simulink library "dtcBswLib"  (R2023b)
settings: Solver=VariableStepAuto  StartTime=0.0  StopTime=10.0  RelTol=1e-3
libraries: dtc_bswapi x5, simulink x2
settings Model: Creator=Professional  LastModifiedBy=zon07
settings SFSimCC: SimAnalyzeCustomCode=on  SimTargetLang=C++
settings RTWCC: RTWUseSimCustomCode=on

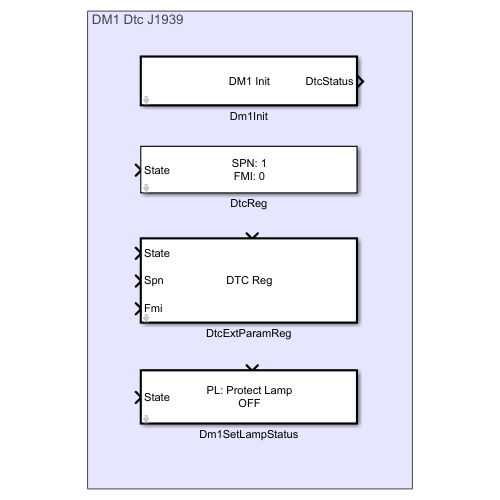
[thumbnail: Simulink's stored preview of the top-level diagram]
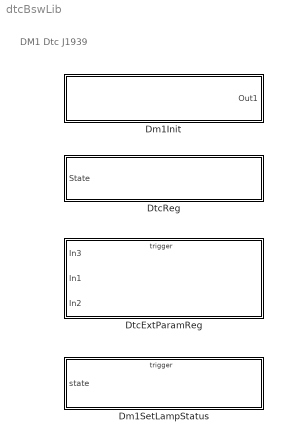
== system dtcBswLib ==
  note: DM1 Dtc J1939
  Dm1Init : Subsystem  TreatAsAtomicUnit=on  mask(Инициализация сервиса DM1){can='CAN1', message_priority='Priority #6', source_address=0x31}
      mask prompts: can "Номер модуля CAN:"; message_priority "Приоритет сообщения:"; source_address "Адрес источника:"
      mask help:
      | Задайте приоритет и адрес источника диагностического сообщения согласно j1939.
      | Status вернет true если будет обнаружена хотя-бы одна неисправность.
      mask TypeOptions can: 'CAN1' | 'CAN2'
      mask Display:
      | disp('DM1 Init');
      | port_label('output', 1, 'DtcStatus');
  Dm1SetLampStatus : Subsystem  mask(DM1 Lamp Status){lamp=PL: Protect Lamp, flash=OFF}
      mask prompts: lamp "Диагностическая лампа:"; flash "Мигание лампы:"
      mask help:
      | Функцию необходимо вызвать.
      | Управление диагностическими лампами.
      |
      | State:
      | 0 - Выключение лампы;
      | 1 - Включение лампы;
      |
      | Комбинации State и Flash согласно J1939.
      mask init:
      | maskObj = Simulink.Mask.get(gcb);
      | lampName = maskObj.getParameter('lamp').Value;
      | flashName = maskObj.getParameter('flash').Value;
      | 
      | blockName = lampName + "\n" + flashName;
      mask TypeOptions lamp: PL: Protect Lamp | AWL: Amber Warning Lamp | RSL: Red Stop Lamp | MIL: Malfunction Indicator Lamp
      mask DialogControl ParameterGroupVar Prompt: Параметры
      mask Display:
      | disp(blockName);
      | port_label('input', 1, 'State');
  DtcExtParamReg : Subsystem  mask(Регистрация Dtc внешними параметрами){}
      mask help:
      | Функцию необходимо вызвать.
      | State - Состояние ошибки: true - активировать, false - деактивировать;
      | Spn - номер Dtc: 0 - 524287;
      | Fmi - код Dtc: 0 - 31;
      mask init:
      | block_name = "DTC Reg";
      mask Display:
      | disp(block_name);
      | port_label('input', 1, 'State');
      | port_label('input', 2, 'Spn');
      | port_label('input', 3, 'Fmi');
  DtcReg : Subsystem  mask(Регистрация Dtc){block_name=0, spn=1, fmi=0}
      mask help:
      | Задайте SPN и FMI ошибки.
      | Ошибка регистрируется по изменению состояния входа State;
      |
      | Состояние ошибки переключиться при изменении значения на входе State.
      | При переходе из false -> true - ошибка активируется;
      | При переходе из true -> false - ошибка деактивируется;
      mask init:
      | block_name = "SPN: " + num2str(spn) + "\nFMI: " + num2str(fmi);
      mask Display:
      | disp(block_name);
      | port_label('input', 1, 'State');

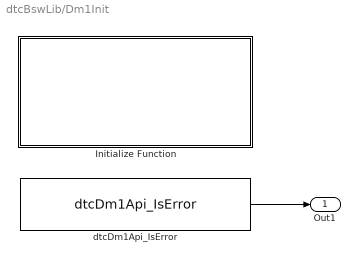
== system dtcBswLib/Dm1Init ==
  Initialize Function : Subsystem  TreatAsAtomicUnit=on
  dtcDm1Api_IsError : dtc_bswapi/dtcDm1Api_IsError  SampleTime=-1
  Out1 : Outport  OutDataTypeStr=boolean
  wires:
  dtcDm1Api_IsError/1 -> Out1/1

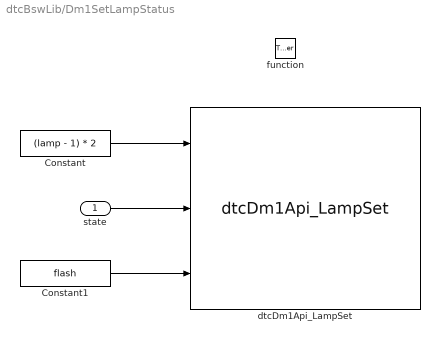
== system dtcBswLib/Dm1SetLampStatus ==
  state : Inport
  function : TriggerPort  TriggerType=function-call  VariantControl=(inherit)
  Constant : Constant  Value=(lamp - 1) * 2  OutDataTypeStr=uint8
  Constant1 : Constant  Value=flash  OutDataTypeStr=uint8
  dtcDm1Api_LampSet : dtc_bswapi/dtcDm1Api_LampSet  SampleTime=-1
  wires:
  Constant/1 -> dtcDm1Api_LampSet/1
  state/1 -> dtcDm1Api_LampSet/2
  Constant1/1 -> dtcDm1Api_LampSet/3

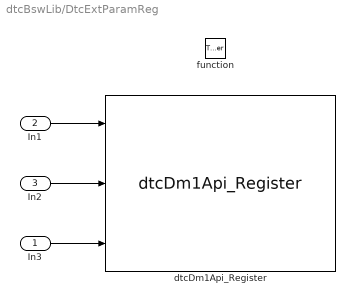
== system dtcBswLib/DtcExtParamReg ==
  In3 : Inport  OutDataTypeStr=boolean
  In1 : Inport  Port=2  OutDataTypeStr=uint32
  In2 : Inport  Port=3  OutDataTypeStr=uint8
  function : TriggerPort  TriggerType=function-call  VariantControl=(inherit)
  dtcDm1Api_Register : dtc_bswapi/dtcDm1Api_Register  SampleTime=-1
  wires:
  In1/1 -> dtcDm1Api_Register/1
  In2/1 -> dtcDm1Api_Register/2
  In3/1 -> dtcDm1Api_Register/3

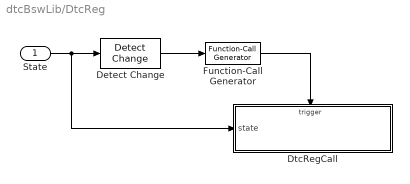
== system dtcBswLib/DtcReg ==
  State : Inport  OutDataTypeStr=boolean
  Detect Change : simulink/Logic and Bit Operations/Detect Change  vinit=0  OutDataTypeStr=boolean
  DtcRegCall : Subsystem  TreatAsAtomicUnit=on
  Function-Call Generator : simulink/Ports & Subsystems/Function-Call Generator  sample_time=1  numberOfIterations=1  DisallowWideOutput=off  ShowEnablePort=on
  wires:
  Function-Call Generator/1 -> DtcRegCall/Trigger
  Detect Change/1 -> Function-Call Generator/1
  State/1 -> DtcRegCall/1(state), Detect Change/1

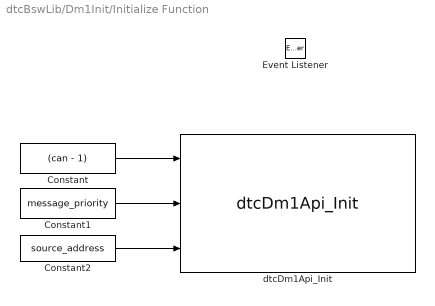
== system dtcBswLib/Dm1Init/Initialize Function ==
  Constant : Constant  Value=(can - 1)  OutDataTypeStr=int32
  Constant1 : Constant  Value=message_priority  OutDataTypeStr=uint8
  Constant2 : Constant  Value=source_address  OutDataTypeStr=uint8
  Event Listener : EventListener  DisableCoverage=on  EventName=reset
  dtcDm1Api_Init : dtc_bswapi/dtcDm1Api_Init  SampleTime=-1
  wires:
  Constant2/1 -> dtcDm1Api_Init/3
  Constant1/1 -> dtcDm1Api_Init/2
  Constant/1 -> dtcDm1Api_Init/1

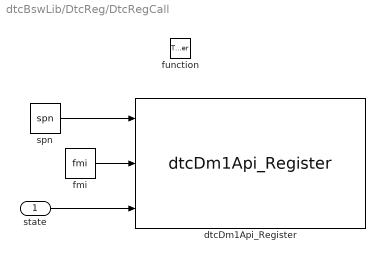
== system dtcBswLib/DtcReg/DtcRegCall ==
  state : Inport
  function : TriggerPort  TriggerType=function-call  VariantControl=(inherit)
  dtcDm1Api_Register : dtc_bswapi/dtcDm1Api_Register  SampleTime=-1
  fmi : Constant  Value=fmi  OutDataTypeStr=uint8
  spn : Constant  Value=spn  OutDataTypeStr=uint32
  wires:
  fmi/1 -> dtcDm1Api_Register/2
  spn/1 -> dtcDm1Api_Register/1
  state/1 -> dtcDm1Api_Register/3
